simulink library "common_lib"  (R2021b)
settings: Solver=ode45  StartTime=0.0  StopTime=10.0  RelTol=1e-3
undefined symbols (not defined in the file or in its folder): ACCEL_PRE_MULT, C_C1GearNumbers, C_C1GearRatios, C_Calibration, C_DitherWaveform, C_GearOffset, C_GearRatioIn, C_GearRatioInverseOut, C_GearRatioOut, CLUTCH_INNER_LOOP_UPDATE_RATE, CONSTANT, DEGRADED_MODE_SIZE, Dem_EventStatusType, DiscIntNeverNeededParam, F_FAULT_ENUM, F_NOFAULT, F_OUTOFRANGE, F_RATELIMIT, FALSE, FMI14_SPECIAL_INSTRUCTIONS, FMI20_DATA_DRIFTED_HIGH, FMI21_DATA_DRIFTED_LOW, FMI29_RESERVED_FOR_SAE_ASSIGNMENT, FMI30_RESERVED_FOR_SAE_ASSIGNMENT, FMI31_CONDITION_EXISTS, FMI32_NO_FAULT, IC, k_accel, k_mean, LVDCU_OORH_FaultCntThd_C, MAX_UINT32, MEAN_PRE_MULT, NTriggers, QLTY_SIGNAL_FAILED, QLTY_SIGNAL_FULLY_FUNCTION, QLTY_SIGNAL_SUBSTITUTED_BY_1ST_CHOICE, QLTY_SIGNAL_SUBSTITUTED_BY_2ND_CHOICE, QLTY_SIGNAL_SUBSTITUTED_BY_3RD_CHOICE, QLTY_SIGNAL_SUBSTITUTED_BY_4TH_CHOICE, SAMPLE_TIME_100_mSec, SAMPLE_TIME_100_uSec, simin, T_TestPoint, TF_FALSE, TF_TRUE, TimeStep, TRUE, WORKSPACE_UPDATE_RATE, ZERO, Zero
libraries: $bdroot x120, simulink x27, simulink_extras x4, MBD_EPS_Local_Blockset x4
(part 8 of 10)

== system common_lib/Slink/Variable Rate Limiter ==
  note: Common Library::Simulink Enhancements::Rate Limiter
  input : Inport
  rise rate : Inport  Port=2
  fall rate : Inport  Port=3
  Data Type Conversion : DataTypeConversion  OutDataTypeStr=single
  Product : Product  InputSameDT=on  OutDataTypeStr=Inherit: Same as first input
  Product1 : Product  Inputs=/*  InputSameDT=on  OutDataTypeStr=Inherit: Same as first input
  Sat : $bdroot/Slink/Sat
  Sum2 : Sum  Inputs=|++  InputSameDT=on  OutDataTypeStr=Inherit: Same as first input
  Sum3 : Sum  Inputs=|+-  InputSameDT=on  OutDataTypeStr=Inherit: Same as first input
  T : Constant  Value=TimeStep
  Unit Delay : UnitDelay  InitialCondition=ic  SampleTime=-1  HasFrameUpgradeWarning=on
  output : Outport  VectorParamsAs1DForOutWhenUnconnected=off
  wires:
  Data Type Conversion/1 -> Product1/1, Product/1
  T/1 -> Data Type Conversion/1
  rise rate/1 -> Sat/2
  fall rate/1 -> Sat/3
  Sum3/1 -> Product1/2
  Product/1 -> Sum2/1
  Sum2/1 -> output/1, Unit Delay/1
  Unit Delay/1 -> Sum2/2, Sum3/2
  Product1/1 -> Sat/1  "Slope"
  input/1 -> Sum3/1
  Sat/1 -> Product/2

== system common_lib/Slink/Variable Rate Limiter w IC ==
  note: Common Library::Simulink Enhancements::Rate Limiter with Reset
  input : Inport
  rise rate : Inport  Port=2
  fall rate : Inport  Port=3
  ic : Inport  Port=4
  reset? : Inport  Port=5  OutDataTypeStr=boolean
  Data Type Conversion : DataTypeConversion  OutDataTypeStr=single
  Product : Product  InputSameDT=on  OutDataTypeStr=Inherit: Same as first input
  Product1 : Product  Inputs=/*  InputSameDT=on  OutDataTypeStr=Inherit: Same as first input
  Sat : $bdroot/Slink/Sat
  Sum2 : Sum  Inputs=|++  InputSameDT=on  OutDataTypeStr=Inherit: Same as first input
  Sum3 : Sum  Inputs=|+-  InputSameDT=on  OutDataTypeStr=Inherit: Same as first input
  Switch2 : Switch  Threshold=0.5  ZeroCross=off  InputSameDT=on
  T : Constant  Value=TimeStep
  Unit Delay1 : UnitDelay  InitialCondition=ic  SampleTime=-1  HasFrameUpgradeWarning=on
  output : Outport  VectorParamsAs1DForOutWhenUnconnected=off
  wires:
  Data Type Conversion/1 -> Product1/1, Product/1
  T/1 -> Data Type Conversion/1
  Switch2/1 -> Unit Delay1/1, output/1
  Sum2/1 -> Switch2/3
  Unit Delay1/1 -> Sum3/2, Sum2/2
  ic/1 -> Switch2/1
  reset?/1 -> Switch2/2
  Sat/1 -> Product/2
  input/1 -> Sum3/1
  Product1/1 -> Sat/1  "Slope"
  Product/1 -> Sum2/1
  Sum3/1 -> Product1/2
  fall rate/1 -> Sat/3
  rise rate/1 -> Sat/2

== system common_lib/Slink/Variable Rate Limiter w IC and Sat ==
  note: Common Library::Simulink Enhancements::Rate Limiter with Reset and Saturation
  input : Inport
  rise rate : Inport  Port=2
  fall rate : Inport  Port=3
  ulim : Inport  Port=4
  llim : Inport  Port=5
  ic : Inport  Port=6
  reset? : Inport  Port=7  OutDataTypeStr=boolean
  Data Type Conversion : DataTypeConversion  OutDataTypeStr=single
  Product : Product  InputSameDT=on  OutDataTypeStr=Inherit: Same as first input
  Product1 : Product  Inputs=/*  InputSameDT=on  OutDataTypeStr=Inherit: Same as first input
  Sat : $bdroot/Slink/Sat
  Sat1 : $bdroot/Slink/Sat
  Sum2 : Sum  Inputs=|++  InputSameDT=on  OutDataTypeStr=Inherit: Same as first input
  Sum3 : Sum  Inputs=|+-  InputSameDT=on  OutDataTypeStr=Inherit: Same as first input
  Switch2 : Switch  Threshold=0.5  ZeroCross=off  InputSameDT=on
  T : Constant  Value=TimeStep
  Unit Delay1 : UnitDelay  InitialCondition=ic  SampleTime=-1  HasFrameUpgradeWarning=on
  output : Outport  VectorParamsAs1DForOutWhenUnconnected=off
  wires:
  Data Type Conversion/1 -> Product1/1, Product/1
  T/1 -> Data Type Conversion/1
  llim/1 -> Sat1/3
  ulim/1 -> Sat1/2
  Switch2/1 -> Sat1/1
  Sat1/1 -> Unit Delay1/1, output/1
  Sum2/1 -> Switch2/3
  Unit Delay1/1 -> Sum3/2, Sum2/2
  ic/1 -> Switch2/1
  reset?/1 -> Switch2/2
  Sat/1 -> Product/2
  input/1 -> Sum3/1
  Product1/1 -> Sat/1  "Slope"
  Product/1 -> Sum2/1
  Sum3/1 -> Product1/2
  fall rate/1 -> Sat/3
  rise rate/1 -> Sat/2

== system common_lib/Tbl/2D Lookup ==
  Input : Inport
  X Axis : Inport  Port=2
  Y Axis : Inport  Port=3
  Mux : Mux  Inputs=3
  S-Function : S-Function  FunctionName=vartable  Parameters=Mode  SFunctionDeploymentMode=off  EnableBusSupport=off
  Output : Outport  VectorParamsAs1DForOutWhenUnconnected=off
  wires:
  Mux/1 -> S-Function/1
  Input/1 -> Mux/1
  X Axis/1 -> Mux/2
  S-Function/1 -> Output/1
  Y Axis/1 -> Mux/3

== system common_lib/Tbl/Interpolator ==
  note: Common Library::Tables::Interpolator
  value_1 : Inport
  value_0 : Inport  Port=2
  interp_factor : Inport  Port=3
  Constant1 : Constant  Value=Zero
  Constant2 : Constant  Value=One
  XY Interpolator : $bdroot/Tbl/XY Interpolator  DType=double
  output : Outport  VectorParamsAs1DForOutWhenUnconnected=off
  wires:
  value_0/1 -> XY Interpolator/2
  value_1/1 -> XY Interpolator/1
  Constant2/1 -> XY Interpolator/3
  Constant1/1 -> XY Interpolator/4
  interp_factor/1 -> XY Interpolator/5
  XY Interpolator/1 -> output/1

== system common_lib/Tbl/XY Interpolator ==
  note: Common Library::Tables::XY Interpolator
  y_value_1 : Inport
  y_value_0 : Inport  Port=2
  x_value_1 : Inport  Port=3
  x_value_0 : Inport  Port=4
  x_value : Inport  Port=5
  Interp : S-Function  FunctionName=xyinterp_f32_wrap  SFunctionModules=xyinterp_f32  SFunctionDeploymentMode=off  EnableBusSupport=off
  output : Outport  VectorParamsAs1DForOutWhenUnconnected=off
  wires:
  y_value_1/1 -> Interp/1
  y_value_0/1 -> Interp/2
  x_value_1/1 -> Interp/3
  x_value_0/1 -> Interp/4
  x_value/1 -> Interp/5
  Interp/1 -> output/1

== system common_lib/Tbl/XY Interpolator1 ==
  note: Common Library::Tables::XY Interpolator
  y_value_1 : Inport
  y_value_0 : Inport  Port=2
  x_value_1 : Inport  Port=3
  x_value_0 : Inport  Port=4
  x_value : Inport  Port=5
  DTC{,1..4} (5 alike) : DataTypeConversion  OutDataTypeStr=single
  Signal Conversion : SignalConversion  ConversionOutput=Contiguous copy  OverrideOpt=on
  XYInterp : Subsystem  TreatAsAtomicUnit=on  RTWFcnName=XYINT
      settings: RTWFcnNameOpts=User specified  RTWFileNameOpts=Use function name
  output : Outport  VectorParamsAs1DForOutWhenUnconnected=off
  wires:
  Signal Conversion/1 -> output/1
  DTC4/1 -> XYInterp/5(x_value)
  DTC3/1 -> XYInterp/4(x_value_0)
  DTC2/1 -> XYInterp/3(x_value_1)
  DTC1/1 -> XYInterp/2(y_value_0)
  DTC/1 -> XYInterp/1(y_value_1)
  x_value/1 -> DTC4/1
  x_value_0/1 -> DTC3/1
  x_value_1/1 -> DTC2/1
  XYInterp/1(output) -> Signal Conversion/1
  y_value_0/1 -> DTC1/1
  y_value_1/1 -> DTC/1

== system common_lib/Timers/Timer ==
  In : Inport
  TriggerTime : Inport  Port=2
  Data Type Conversion : DataTypeConversion  OutDataTypeStr=single
  Discrete-Time Integrator : DiscreteIntegrator  gainval=single(1.0)  ExternalReset=falling  InitialCondition=single(0)  SampleTime=TimeStep  LimitOutput=on  ICPrevOutput=DiscIntNeverNeededParam  ICPrevScaledInput=DiscIntNeverNeededParam
  Relational Operator : RelationalOperator  Operator=>  OutDataTypeStr=boolean  RndMeth=Nearest
  Signal Specification : SignalSpecification  OutDataTypeStr=boolean
  Out : Outport  VectorParamsAs1DForOutWhenUnconnected=off
  wires:
  Signal Specification/1 -> Discrete-Time Integrator/2, Data Type Conversion/1
  In/1 -> Signal Specification/1
  Data Type Conversion/1 -> Discrete-Time Integrator/1
  Discrete-Time Integrator/1 -> Relational Operator/1
  TriggerTime/1 -> Relational Operator/2
  Relational Operator/1 -> Out/1

== system common_lib/Approved Simulink/Basic IO/M_MonitorParameter1 ==
  Input : Inport
  towork : ToWorkspace  VariableName=ToWorkspace  SampleTime=-1
      settings: Description=Monitor  Decimation=WORKSPACE_DECIMATION
  wires:
  Input/1 -> towork/1  "ToWorkspace"

== system common_lib/Approved Simulink/Basic IO/To xPC Scope1 ==
  Inport : Inport
  Terminate : Terminator
  wires:
  Inport/1 -> Terminate/1

== system common_lib/Approved Simulink/SubSys Triggers/Configurable Subsystem ==

== system common_lib/Approved Simulink/SubSys Triggers/For Iterator Subsystem ==
  In1 : Inport
  For Iterator : ForIterator
  Out1 : Outport  VectorParamsAs1DForOutWhenUnconnected=off
  wires:
  In1/1 -> Out1/1

== system common_lib/Approved Simulink/SubSys Triggers/If Action Subsystem ==
  In1 : Inport
  Action Port : ActionPort
  Out1 : Outport  VectorParamsAs1DForOutWhenUnconnected=off
  wires:
  In1/1 -> Out1/1

== system common_lib/Approved Simulink/SubSys Triggers/Subsystem ==
  In1 : Inport
  Out1 : Outport  VectorParamsAs1DForOutWhenUnconnected=off
  wires:
  In1/1 -> Out1/1

== system common_lib/Approved Simulink/SubSys Triggers/While Iterator Subsystem ==
  In1 : Inport
  IC : Inport  Port=2
  While Iterator : WhileIterator
  Out1 : Outport  VectorParamsAs1DForOutWhenUnconnected=off
  wires:
  IC/1 -> While Iterator/2
  In1/1 -> Out1/1

== system common_lib/Ctrl/DTNA_PIgov/Integrator ==
  note: Common Library::Integral
  input : Inport
  ulim : Inport  Port=2
  llim : Inport  Port=3
  ic : Inport  Port=4
  reset? : Inport  Port=5  OutDataTypeStr=boolean
  Constant1 : Constant  Value=TimeStep  OutDataTypeStr=Inherit: Inherit via back propagation
  Product1 : Product  Inputs=**  InputSameDT=on  OutDataTypeStr=Inherit: Same as first input
  Sat : Subsystem  AncestorBlock=common_lib/Slink/Sat  mask(CL Variable Saturation){}
      mask help:
      | Variable saturation block
      |
      | X(1) = input
      | X(2) = upper limit
      | X(3) = lower limit
      |
      | Y(1) = output
      | NgEK, Inc.
      mask Help: web(which(['common_lib37.html']))
      mask Display:
      | patch([0.3 0.3 0.7 0.7], [0.35 0.65 0.65 0.35], [255/255 127/255 255/255])
      | 
      | plot([0 1],[0.5 0.5],[0.5 0.5],[0 1],[0 0.25 0.75 1],[0 0 1 1])
  Sum : Sum  Inputs=++|  InputSameDT=on  OutDataTypeStr=Inherit: Same as first input
  Switch : Switch  Threshold=0.5  ZeroCross=off  InputSameDT=on
  Unit Delay : UnitDelay  InitialCondition=IC  SampleTime=-1  HasFrameUpgradeWarning=on
  Output : Outport  VectorParamsAs1DForOutWhenUnconnected=off
  wires:
  Constant1/1 -> Product1/1
  Sat/1(output) -> Unit Delay/1, Output/1
  Unit Delay/1 -> Sum/1
  Switch/1 -> Sat/1(input)
  Sum/1 -> Switch/3
  llim/1 -> Sat/3(llim)
  ulim/1 -> Sat/2(ulim)
  reset?/1 -> Switch/2
  Product1/1 -> Sum/2
  ic/1 -> Switch/1
  input/1 -> Product1/2

== system common_lib/Ctrl/Derivative/DerivativeCoreLogic ==
  note: s
      | H(s) = ----------------
      |              1+s/Klo
  note: Derivative Filter Obtained By Backward Differencing Of
  input : Inport  OutDataTypeStr=single
  cutoff : Inport  Port=2  OutDataTypeStr=single
  reset? : Inport  Port=3  OutDataTypeStr=boolean
  ulim : Inport  Port=4
  llim : Inport  Port=5
  Constant1 : Constant  Value=One
  Constant6 : Constant  Value=Zero
  IC:  0 : UnitDelay  InitialCondition=Zero  SampleTime=-1  HasFrameUpgradeWarning=on
  IC: 0 : UnitDelay  InitialCondition=Zero  SampleTime=-1  HasFrameUpgradeWarning=on
  Product2 : Product  Inputs=*/  InputSameDT=on  OutDataTypeStr=Inherit: Same as first input
  Sat : $bdroot/Slink/Sat
  Sum : Sum  Inputs=++-  InputSameDT=on  OutDataTypeStr=Inherit: Same as first input
  Sum3 : Sum  Inputs=|++  InputSameDT=on  OutDataTypeStr=Inherit: Same as first input
  Switch : Switch  Criteria=u2 ~= 0  Threshold=0.5  ZeroCross=off  InputSameDT=on
  output : Outport  OutDataTypeStr=single  VectorParamsAs1DForOutWhenUnconnected=off
  wires:
  reset?/1 -> Switch/2
  Switch/1 -> IC: 0/1, Sat/1
  Constant6/1 -> Switch/1
  Product2/1 -> Switch/3
  IC: 0/1 -> Sum/1
  Sum3/1 -> Product2/2
  Constant1/1 -> Sum3/2
  IC:  0/1 -> Sum/3
  input/1 -> IC:  0/1, Sum/2
  cutoff/1 -> Sum3/1
  Sum/1 -> Product2/1
  ulim/1 -> Sat/2
  llim/1 -> Sat/3
  Sat/1 -> output/1

== system common_lib/Ctrl/PIgov/Integrator01 ==
  note: Common Library::Integral
  input : Inport
  ulim : Inport  Port=2
  llim : Inport  Port=3
  ic : Inport  Port=4
  reset? : Inport  Port=5  OutDataTypeStr=boolean
  Constant1 : Constant  Value=TimeStep
  Product1 : Product  Inputs=**  InputSameDT=on  OutDataTypeStr=Inherit: Same as first input
  Sat : $bdroot/Slink/Sat
  Sum : Sum  Inputs=++|  InputSameDT=on  OutDataTypeStr=Inherit: Same as first input
  Switch : Switch  Threshold=0.5  ZeroCross=off  InputSameDT=on
  Unit Delay : UnitDelay  InitialCondition=IC  SampleTime=-1  HasFrameUpgradeWarning=on
  Output : Outport  VectorParamsAs1DForOutWhenUnconnected=off
  wires:
  Constant1/1 -> Product1/1
  Sat/1 -> Unit Delay/1, Output/1
  Unit Delay/1 -> Sum/1
  Switch/1 -> Sat/1
  Sum/1 -> Switch/3
  llim/1 -> Sat/3
  ulim/1 -> Sat/2
  reset?/1 -> Switch/2
  Product1/1 -> Sum/2
  ic/1 -> Switch/1
  input/1 -> Product1/2

== system common_lib/Ctrl/Trajectory/CurrentStart ==
  in : Inport
  Enable : EnablePort  ZeroCross=off
  out : Outport  VectorParamsAs1DForOutWhenUnconnected=off
  wires:
  in/1 -> out/1

== system common_lib/Ctrl/Trajectory/Start ==
  in : Inport
  Enable : EnablePort  ZeroCross=off
  out : Outport  VectorParamsAs1DForOutWhenUnconnected=off
  wires:
  in/1 -> out/1

== system common_lib/Ctrl/Trajectory/Variable Rate Limiter w IC in feedback loop ==
  note: Common Library::Simulink Enhancements::Rate Limiter with IC in feedback loop
  input : Inport
  rise rate : Inport  Port=2
  fall rate : Inport  Port=3
  ic : Inport  Port=4
  reset? : Inport  Port=5  OutDataTypeStr=boolean
  Product : Product  InputSameDT=on  OutDataTypeStr=Inherit: Same as first input
  Product1 : Product  Inputs=/*  InputSameDT=on  OutDataTypeStr=Inherit: Same as first input
  Sat : $bdroot/Slink/Sat
  Sum2 : Sum  Inputs=|++  InputSameDT=on  OutDataTypeStr=Inherit: Same as first input
  Sum3 : Sum  Inputs=|+-  InputSameDT=on  OutDataTypeStr=Inherit: Same as first input
  Switch2 : Switch  Threshold=0.5  ZeroCross=off  InputSameDT=on
  T : Constant  Value=TimeStep
  Unit Delay1 : UnitDelay  InitialCondition=ic  SampleTime=-1  HasFrameUpgradeWarning=on
  output : Outport  VectorParamsAs1DForOutWhenUnconnected=off
  wires:
  Switch2/1 -> Sum2/2, Sum3/2
  input/1 -> Sum3/1
  Sum2/1 -> Unit Delay1/1, output/1
  Unit Delay1/1 -> Switch2/3
  ic/1 -> Switch2/1
  reset?/1 -> Switch2/2
  Sat/1 -> Product/2
  Product1/1 -> Sat/1  "Slope"
  Product/1 -> Sum2/1
  Sum3/1 -> Product1/2
  T/1 -> Product1/1, Product/1
  fall rate/1 -> Sat/3
  rise rate/1 -> Sat/2

== system common_lib/Diag/Command Feedback Test/CommandFeedbackFaultLogicCore ==
  note: Check for command-feedback error exceeding threshold.
  note: Check for "steady state"
  cmd : Inport  OutDataTypeStr=single
  fbk : Inport  Port=2  OutDataTypeStr=single
  tau : Inport  Port=3  OutDataTypeStr=single
  tau_lim : Inport  Port=4  OutDataTypeStr=single
  tau_time : Inport  Port=5  OutDataTypeStr=single
  error_lim : Inport  Port=6  OutDataTypeStr=single
  error_time : Inport  Port=7  OutDataTypeStr=single
  Abs : Abs  ZeroCross=off
  Abs2 : Abs  ZeroCross=off
  Constant1 : Constant  Value=Zero
  Constant3 : Constant  Value=Zero
  Constant5 : Constant  Value=MinusOne
  EdgeTriggered Pulse w/time1 : $bdroot/Misc/EdgeTriggered Pulse w time  Edge=TRUE to FALSE  Pulse=TRUE  TimeStep=TimeStep  Init=0
  Fltr : $bdroot/Fltrs/Fltr  TimeStep=TimeStep
  Latch : $bdroot/Misc/Latch  IC=false
  Logical Operator1 : Logic  Operator=OR
  Product2 : Product  InputSameDT=on  OutDataTypeStr=Inherit: Same as first input
  Relational Operator1 : RelationalOperator  ZeroCross=off  RndMeth=Nearest  InputSameDT=on
  Relational Operator2 : RelationalOperator  ZeroCross=off  RndMeth=Nearest  InputSameDT=on
  Relational Operator3 : RelationalOperator  ZeroCross=off  RndMeth=Nearest  InputSameDT=on
  Relational Operator4 : RelationalOperator  Operator=<=  ZeroCross=off  RndMeth=Nearest  InputSameDT=on
  Sat : $bdroot/Slink/Sat
  Sum : Sum  Inputs=|+-  InputSameDT=on  OutDataTypeStr=Inherit: Same as first input
  Sum2 : Sum  Inputs=|+-  InputSameDT=on  OutDataTypeStr=Inherit: Same as first input
  Sum3 : Sum  Inputs=++|  InputSameDT=on  OutDataTypeStr=Inherit: Same as first input
  T1 : Constant  Value=Ts
  Unit Delay1 : UnitDelay  InitialCondition=Zero  SampleTime=-1  HasFrameUpgradeWarning=on
  dec switch : Switch  Threshold=0.5  ZeroCross=off  InputSameDT=on
  dec switch1 : Switch  Threshold=0.5  ZeroCross=off  InputSameDT=on
  Min Value : Outport  OutDataTypeStr=boolean  VectorParamsAs1DForOutWhenUnconnected=off
  wires:
  T1/1 -> Product2/1, dec switch1/1
  Product2/1 -> dec switch1/3
  Constant5/1 -> Product2/2
  Relational Operator4/1 -> Latch/2
  Relational Operator3/1 -> Latch/1
  Latch/1 -> Min Value/1
  Logical Operator1/1 -> dec switch/2
  Relational Operator2/1 -> dec switch1/2
  Constant1/1 -> dec switch/1
  dec switch1/1 -> dec switch/3
  Unit Delay1/1 -> Sum3/1
  Sat/1 -> Unit Delay1/1
  dec switch/1 -> Sum3/2
  Constant3/1 -> Relational Operator4/2, Sat/3
  error_time/1 -> Relational Operator3/2, Sat/2
  Sum3/1 -> Relational Operator4/1, Relational Operator3/1, Sat/1
  error_lim/1 -> Relational Operator2/2
  Abs/1 -> Relational Operator2/1
  EdgeTriggered Pulse w/time1/1 -> Logical Operator1/2
  tau_time/1 -> EdgeTriggered Pulse w/time1/2
  Relational Operator1/1 -> Logical Operator1/1, EdgeTriggered Pulse w/time1/1
  tau_lim/1 -> Relational Operator1/2
  Abs2/1 -> Relational Operator1/1
  Sum2/1 -> Abs2/1
  tau/1 -> Fltr/2
  Fltr/1 -> Sum2/2
  Sum/1 -> Abs/1
  fbk/1 -> Sum/2
  cmd/1 -> Sum2/1, Fltr/1, Sum/1

== system common_lib/Diag/Fault Counter/FaultCounter ==
  fl : Inport
  count_prev : Inport  Port=2
  fc_level : Inport  Port=3
  reset : Inport  Port=4  OutDataTypeStr=boolean
  Enable : EnablePort  ZeroCross=off
  Constant1 : Constant  Value=ZERO
  Constant2 : Constant  Value=false
  Constant3 : Constant  Value=true
  Constant6 : Constant  Value=ZERO
  Relay : $bdroot/Slink/Relay  init=false
      settings: AttributesFormatString=ic=%<init>
  Sat : $bdroot/Slink/Sat
  Sum : Sum  Inputs=++|  InputSameDT=on  OutDataTypeStr=Inherit: Same as first input
  reset switch1 : Switch  Criteria=u2 ~= 0  Threshold=0.5  ZeroCross=off  InputSameDT=on
  count : Outport  OutputWhenDisabled=reset  InitialOutput=ZERO  VectorParamsAs1DForOutWhenUnconnected=off
  fc : Outport  Port=2  OutputWhenDisabled=reset  InitialOutput=false  VectorParamsAs1DForOutWhenUnconnected=off
  wires:
  Sum/1 -> reset switch1/3
  Constant6/1 -> reset switch1/1
  Relay/1 -> fc/1
  Constant3/1 -> Relay/4
  Constant2/1 -> Relay/5
  Constant1/1 -> Relay/3, Sat/3
  fc_level/1 -> Relay/2, Sat/2
  fl/1 -> Sum/2
  reset/1 -> reset switch1/2
  reset switch1/1 -> Relay/1, Sat/1
  count_prev/1 -> Sum/1
  Sat/1 -> count/1

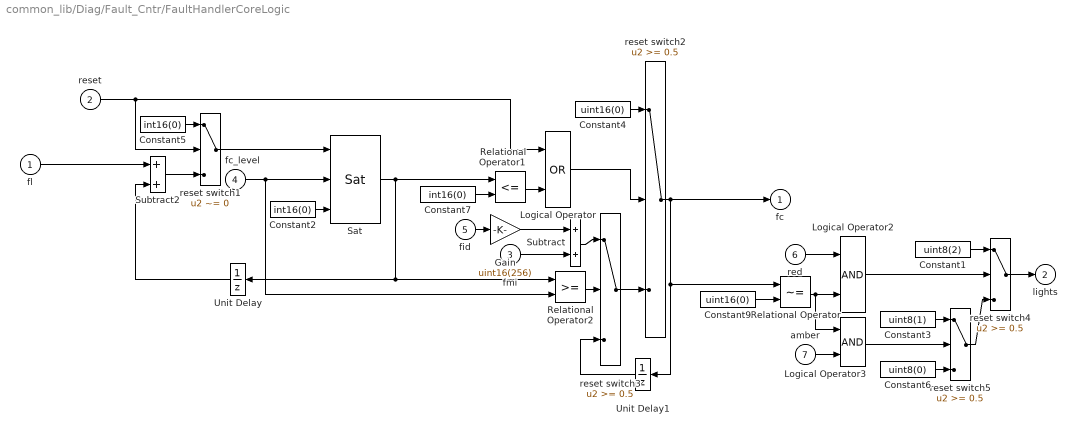
== system common_lib/Diag/Fault_Cntr/FaultHandlerCoreLogic ==
  fl : Inport  OutDataTypeStr=int16
  reset : Inport  Port=2  OutDataTypeStr=boolean
  fmi : Inport  Port=3  OutDataTypeStr=uint16
  fc_level : Inport  Port=4  OutDataTypeStr=int16
  fid : Inport  Port=5  OutDataTypeStr=uint16
  red : Inport  Port=6  OutDataTypeStr=boolean
  amber : Inport  Port=7  OutDataTypeStr=boolean
  Constant1 : Constant  Value=uint8(2)
  Constant2 : Constant  Value=int16(0)
  Constant3 : Constant  Value=uint8(1)
  Constant4 : Constant  Value=uint16(0)
  Constant5 : Constant  Value=int16(0)
  Constant6 : Constant  Value=uint8(0)
  Constant7 : Constant  Value=int16(0)
  Constant9 : Constant  Value=uint16(0)
  Gain : Gain  Gain=uint16(256)
  Logical Operator : Logic  Operator=OR  AllPortsSameDT=off  OutDataTypeStr=boolean
  Logical Operator2 : Logic  AllPortsSameDT=off  OutDataTypeStr=boolean
  Logical Operator3 : Logic  AllPortsSameDT=off  OutDataTypeStr=boolean
  Relational Operator : RelationalOperator  Operator=~=  OutDataTypeStr=boolean  RndMeth=Nearest
  Relational Operator1 : RelationalOperator  Operator=<=  OutDataTypeStr=boolean  RndMeth=Nearest
  Relational Operator2 : RelationalOperator  OutDataTypeStr=boolean  RndMeth=Nearest
  Sat : $bdroot/Slink/Sat
  Subtract : Sum  OutDataTypeStr=uint16
  Subtract2 : Sum  OutDataTypeStr=int16  SaturateOnIntegerOverflow=on
  Unit Delay : UnitDelay  InitialCondition=int16(0)  SampleTime=-1  HasFrameUpgradeWarning=on
      settings: AttributesFormatString=ic=%<X0>
  Unit Delay1 : UnitDelay  InitialCondition=uint16(0)  SampleTime=-1  HasFrameUpgradeWarning=on
      settings: AttributesFormatString=ic=%<X0>
  reset switch1 : Switch  Criteria=u2 ~= 0  Threshold=0.5  ZeroCross=off  InputSameDT=on
  reset switch{2..5} (4 alike) : Switch  Threshold=0.5  ZeroCross=off  InputSameDT=on
  fc : Outport  VectorParamsAs1DForOutWhenUnconnected=off
  lights : Outport  Port=2  VectorParamsAs1DForOutWhenUnconnected=off
  wires:
  Gain/1 -> Subtract/1
  reset switch3/1 -> reset switch2/3
  Unit Delay1/1 -> reset switch3/3
  Relational Operator2/1 -> reset switch3/2
  Relational Operator1/1 -> Logical Operator/2
  Constant7/1 -> Relational Operator1/2
  Unit Delay/1 -> Subtract2/2
  Subtract2/1 -> reset switch1/3
  reset switch1/1 -> Sat/1
  Constant5/1 -> reset switch1/1
  reset switch2/1 -> Unit Delay1/1, Relational Operator/1, fc/1
  Logical Operator/1 -> reset switch2/2
  Subtract/1 -> reset switch3/1
  Constant4/1 -> reset switch2/1
  fmi/1 -> Subtract/2
  fid/1 -> Gain/1
  reset/1 -> Logical Operator/1, reset switch1/2
  fl/1 -> Subtract2/1
  Sat/1 -> Relational Operator2/1, Unit Delay/1, Relational Operator1/1
  Constant9/1 -> Relational Operator/2
  Logical Operator2/1 -> reset switch4/2
  Relational Operator/1 -> Logical Operator2/2, Logical Operator3/1
  red/1 -> Logical Operator2/1
  amber/1 -> Logical Operator3/2
  fc_level/1 -> Sat/2, Relational Operator2/2
  Constant2/1 -> Sat/3
  Constant1/1 -> reset switch4/1
  Logical Operator3/1 -> reset switch5/2
  reset switch5/1 -> reset switch4/3
  Constant3/1 -> reset switch5/1
  Constant6/1 -> reset switch5/3
  reset switch4/1 -> lights/1

== system common_lib/Diag/Filter w Fault Handler/FilterWithFaultHandlerCoreLogic ==
  note: Common Library::Diagnostics::Filter With Fault Handler
  input : Inport
  tau : Inport  Port=2
  override_value : Inport  Port=3
  override? : Inport  Port=4
  reset? : Inport  Port=5
  default : Inport  Port=6
  ramp_time : Inport  Port=7
  fault? : Inport  Port=8
  Abs1 : Abs  ZeroCross=off
  Abs2 : Abs  ZeroCross=off
  Constant5 : Constant  Value=TimeStep
  Data Type Conversion : DataTypeConversion  OutDataTypeStr=single
  Fltr_wRO : $bdroot/Fltrs/Fltr_wRO  TimeStep=TimeStep
  Product1 : Product  Inputs=**/  InputSameDT=on  OutDataTypeStr=Inherit: Same as first input
  Sum1 : Sum  Inputs=+-|  InputSameDT=on  OutDataTypeStr=Inherit: Same as first input
  Sum2 : Sum  Inputs=+-|  InputSameDT=on  OutDataTypeStr=Inherit: Same as first input
  Sum3 : Sum  Inputs=+-|  InputSameDT=on  OutDataTypeStr=Inherit: Same as first input
  Switch{1..4} (4 alike) : Switch  Threshold=0.5  ZeroCross=off  InputSameDT=on
  delay : UnitDelay  InitialCondition=Zero  SampleTime=-1  HasFrameUpgradeWarning=on
  ic: signal at fault : UnitDelay  InitialCondition=Zero  SampleTime=-1  HasFrameUpgradeWarning=on
  within zero tol of corrections : RelationalOperator  Operator=<  ZeroCross=off  RndMeth=Nearest
  output : Outport  VectorParamsAs1DForOutWhenUnconnected=off
  wires:
  Data Type Conversion/1 -> Product1/2
  Constant5/1 -> Data Type Conversion/1
  Sum3/1 -> Abs1/1
  delay/1 -> Switch2/1
  Switch3/1 -> delay/1
  within zero tol of corrections/1 -> Switch3/2
  Abs2/1 -> within zero tol of corrections/1
  Abs1/1 -> within zero tol of corrections/2
  Sum2/1 -> Switch3/1
  Switch1/1 -> Sum3/1, Sum2/1
  Switch4/1 -> Switch1/3, Sum1/1, ic: signal at fault/1
  ic: signal at fault/1 -> Switch4/1
  Product1/1 -> Abs2/1, Sum2/2
  Sum1/1 -> Product1/1
  default/1 -> Sum3/2, Switch3/3, Sum1/2
  Fltr_wRO/1 -> Switch4/3, output/1
  input/1 -> Switch2/3
  Switch2/1 -> Switch1/1, Fltr_wRO/1
  reset?/1 -> Fltr_wRO/5
  override?/1 -> Fltr_wRO/4
  override_value/1 -> Fltr_wRO/3
  tau/1 -> Fltr_wRO/2
  fault?/1 -> Switch1/2, Switch4/2, Switch2/2
  ramp_time/1 -> Product1/3

== system common_lib/Diag/Filter w Fault Handler1/Fltr_wRO ==
  note: This is a simple 1st order filter block with reset and override.
      |
      |      If override is true (1) then output=override_value
      |      If       reset is true (1) then output=input
      |    otherwise output = previous output + (input - previous output) * T/tau
  note: Common Library::Filters::Filter with Reset and Override
  input : Inport
  tau : Inport  Port=2
  reset? : Inport  Port=3  OutDataTypeStr=boolean
  Constant1 : Constant  Value=TimeStep
  Constant3 : Constant  Value=TimeStep
  MinMax : MinMax  Function=max  Inputs=2  InputSameDT=on  SaturateOnIntegerOverflow=on  ZeroCross=off
  Product : Product  Inputs=**/  InputSameDT=on  OutDataTypeStr=Inherit: Same as first input
  Sum : Sum  Inputs=|+-  InputSameDT=on  OutDataTypeStr=Inherit: Same as first input
  Sum1 : Sum  Inputs=|++  InputSameDT=on  OutDataTypeStr=Inherit: Same as first input
  Switch2 : Switch  Threshold=0.5  ZeroCross=off  InputSameDT=on
  Unit Delay : UnitDelay  InitialCondition=IC  SampleTime=-1  HasFrameUpgradeWarning=on
  output : Outport  VectorParamsAs1DForOutWhenUnconnected=off
  wires:
  Sum1/1 -> Switch2/3
  Product/1 -> Sum1/1
  tau/1 -> MinMax/2
  Constant1/1 -> MinMax/1
  Unit Delay/1 -> Sum1/2, Sum/2
  input/1 -> Switch2/1, Sum/1
  Constant3/1 -> Product/2
  MinMax/1 -> Product/3
  reset?/1 -> Switch2/2
  Sum/1 -> Product/1
  Switch2/1 -> Unit Delay/1, output/1

== system common_lib/Diagnostics/Calibration Enabled Debounce Boolean Input/DiagFaultCounter ==
  diagFaultActive : Inport
  diagStartUpComp : Inport  Port=2
  diagReset : Inport  Port=3
  diagEnable : Inport  Port=4
  diagDbncEnab : Inport  Port=5
  diagFaultCntThresh : Inport  Port=6
  diagPassCntThresh : Inport  Port=7
  diagUpCnt : Inport  Port=8
  diagDnCnt : Inport  Port=9
  diagHealEn : Inport  Port=10
  DiagFaulCounter : Stateflow chart  TreatAsAtomicUnit=on
  diagFaultStatus : Outport  OutputWhenDisabled=reset  InitialOutput=Dem_EventStatusType.DEM_EVENT_STATUS_INIT  VectorParamsAs1DForOutWhenUnconnected=off
  diagFaultCnt : Outport  Port=2  OutputWhenDisabled=reset  InitialOutput=Dem_EventStatusType.DEM_EVENT_STATUS_INIT  VectorParamsAs1DForOutWhenUnconnected=off
  wires:
  diagFaultActive/1 -> DiagFaulCounter/1(diagFaultActive)
  diagFaultCntThresh/1 -> DiagFaulCounter/6(diagFaultCntThresh)
  diagReset/1 -> DiagFaulCounter/3(diagReset)
  diagUpCnt/1 -> DiagFaulCounter/8(diagUpCnt)
  diagDnCnt/1 -> DiagFaulCounter/9(diagDnCnt)
  diagEnable/1 -> DiagFaulCounter/4(diagEnable)
  DiagFaulCounter/1(diagFaultStatus) -> diagFaultStatus/1
  diagDbncEnab/1 -> DiagFaulCounter/5(diagDbncEnab)
  diagStartUpComp/1 -> DiagFaulCounter/2(diagStartUpComp)
  diagPassCntThresh/1 -> DiagFaulCounter/7(diagPassCntThresh)
  diagHealEn/1 -> DiagFaulCounter/10(diagHealEn)
  DiagFaulCounter/2(diagFaultCnt) -> diagFaultCnt/1

== system common_lib/Diagnostics/Calibration Enabled MinMax OOR/Enabled OOR ==
  In : Inport
  ULim : Inport  Port=2
  LLim : Inport  Port=3
  Ext_Fault : Inport  Port=4
  Enable : EnablePort  ZeroCross=off
      settings: AttributesFormatString=%<StatesWhenEnabling>
  Calibration with Pretty Print Value : $bdroot/IO/Calibration with Pretty Print Value  CalValue=C_IMgmt_OOR_MinMaxCapture_Enable  scaling=None
  OOR Fault Detection : $bdroot/Diag/OOR Fault Detection  InitialValue=InitialValue
  OOR MinMax Capture : Subsystem
  Out : Outport  InitialOutput=0  VectorParamsAs1DForOutWhenUnconnected=off
      settings: AttributesFormatString=|
      | OutputWhenDisabled=%<OutputWhenDisabled>
      | InitialOutput=%<InitialOutput>
  Fault : Outport  Port=2  InitialOutput=0  VectorParamsAs1DForOutWhenUnconnected=off
      settings: AttributesFormatString=|
      | OutputWhenDisabled=%<OutputWhenDisabled>
      | InitialOutput=%<InitialOutput>
  Max : Outport  Port=3  VectorParamsAs1DForOutWhenUnconnected=off
      settings: AttributesFormatString=|
      | OutputWhenDisabled=%<OutputWhenDisabled>
      | InitialOutput=%<InitialOutput>
  Min : Outport  Port=4  VectorParamsAs1DForOutWhenUnconnected=off
      settings: AttributesFormatString=|
      | OutputWhenDisabled=%<OutputWhenDisabled>
      | InitialOutput=%<InitialOutput>
  wires:
  LLim/1 -> OOR Fault Detection/3
  ULim/1 -> OOR Fault Detection/2
  In/1 -> OOR Fault Detection/1, OOR MinMax Capture/1(Input)
  Ext_Fault/1 -> OOR Fault Detection/4, OOR MinMax Capture/2(Hold)
  OOR Fault Detection/1 -> Out/1
  OOR Fault Detection/2 -> Fault/1
  OOR MinMax Capture/1(Max) -> Max/1
  OOR MinMax Capture/2(Min) -> Min/1
  Calibration with Pretty Print Value/1 -> OOR MinMax Capture/Enable

== system common_lib/Diagnostics/Calibration Enabled MinMax RLim/Enabled RLim ==
  In : Inport
  RLim : Inport  Port=2
  Ext_Fault : Inport  Port=3
  Enable : EnablePort  ZeroCross=off
      settings: AttributesFormatString=%<StatesWhenEnabling>
  Calibration with Pretty Print Value : $bdroot/IO/Calibration with Pretty Print Value  CalValue=C_IMgmt_RLim_MinMaxCapture_Enable  scaling=None
  Data Type Conversion : DataTypeConversion  OutDataTypeStr=single
  Data Type Conversion1 : DataTypeConversion  OutDataTypeStr=single
  RLim MinMax Capture : Subsystem
  RateLimit : Subsystem  mask{IC=IC, TimeStep=TimeStep}
      mask prompts: IC "Initial Condition"; TimeStep "Update Time"
  out : Outport  VectorParamsAs1DForOutWhenUnconnected=off
      settings: AttributesFormatString=|
      | OutputWhenDisabled=%<OutputWhenDisabled>
      | InitialOutput=%<InitialOutput>
  fault? : Outport  Port=2  VectorParamsAs1DForOutWhenUnconnected=off
      settings: AttributesFormatString=|
      | OutputWhenDisabled=%<OutputWhenDisabled>
      | InitialOutput=%<InitialOutput>
  Max Pos Rate : Outport  Port=3  VectorParamsAs1DForOutWhenUnconnected=off
      settings: AttributesFormatString=|
      | OutputWhenDisabled=%<OutputWhenDisabled>
      | InitialOutput=%<InitialOutput>
  Max Neg Rate : Outport  Port=4  VectorParamsAs1DForOutWhenUnconnected=off
      settings: AttributesFormatString=|
      | OutputWhenDisabled=%<OutputWhenDisabled>
      | InitialOutput=%<InitialOutput>
  wires:
  In/1 -> Data Type Conversion/1, RLim MinMax Capture/1(Input)
  Ext_Fault/1 -> RLim MinMax Capture/2(Hold), RateLimit/3(ext_fault?)
  RateLimit/1(out) -> out/1
  RLim/1 -> Data Type Conversion1/1
  RateLimit/2(fault?) -> fault?/1
  RLim MinMax Capture/2(Min) -> Max Neg Rate/1
  RLim MinMax Capture/1(Max) -> Max Pos Rate/1
  Data Type Conversion/1 -> RateLimit/1(in)
  Data Type Conversion1/1 -> RateLimit/2(rlim)
  Calibration with Pretty Print Value/1 -> RLim MinMax Capture/Enable

== system common_lib/Diagnostics/DTNA_Diag/CC_Diag ==
  diagInput : Inport
  diagStartUpComp : Inport  Port=2
  diagUpCnt : Inport  Port=3
  diagDnCnt : Inport  Port=4
  diagFaultCntThresh : Inport  Port=5
  diagPassCntThresh : Inport  Port=6
  diagDbncEnab : Inport  Port=7
  diagReset : Inport  Port=8
  diagEnable : Inport  Port=9
  diagHealEn : Inport  Port=10
  Ccaller_DiagLv1 : Subsystem  AncestorBlock=common_lib/Diagnostics/Ccaller_DiagLv1  TreatAsAtomicUnit=on
      settings: RTWSystemCode=Nonreusable function
  diagFaultStatus : Outport
  diagFaultCnt : Outport  Port=2
  wires:
  diagInput/1 -> Ccaller_DiagLv1/1(diagFaultActive)
  diagStartUpComp/1 -> Ccaller_DiagLv1/2(diagStartUpComp)
  diagUpCnt/1 -> Ccaller_DiagLv1/8(diagUpCnt)
  diagDnCnt/1 -> Ccaller_DiagLv1/9(diagDnCnt)
  diagFaultCntThresh/1 -> Ccaller_DiagLv1/6(diagFaultCntThresh)
  diagPassCntThresh/1 -> Ccaller_DiagLv1/7(diagPassCntThresh)
  diagDbncEnab/1 -> Ccaller_DiagLv1/5(diagDbncEnable)
  diagReset/1 -> Ccaller_DiagLv1/3(diagReset)
  diagEnable/1 -> Ccaller_DiagLv1/4(diagEnable)
  diagHealEn/1 -> Ccaller_DiagLv1/10(diagHealEn)
  Ccaller_DiagLv1/1(diagFaultStatus) -> diagFaultStatus/1
  Ccaller_DiagLv1/2(diagFaultCnt) -> diagFaultCnt/1

== system common_lib/Diagnostics/DTNA_Diag/S_Diag ==
  diagInput : Inport
  diagStartUpComp : Inport  Port=2
  diagUpCnt : Inport  Port=3
  diagDnCnt : Inport  Port=4
  diagFaultCntThresh : Inport  Port=5
  diagPassCntThresh : Inport  Port=6
  diagDbncEnab : Inport  Port=7
  diagReset : Inport  Port=8
  diagEnable : Inport  Port=9
  diagHealEn : Inport  Port=10
  DiagFaultCounter : Subsystem
  diagFaultStatus : Outport  OutputWhenDisabled=reset  InitialOutput=Dem_EventStatusType.DEM_EVENT_STATUS_INIT  VectorParamsAs1DForOutWhenUnconnected=off
  diagFaultCnt : Outport  Port=2  OutputWhenDisabled=reset  InitialOutput=Dem_EventStatusType.DEM_EVENT_STATUS_INIT  VectorParamsAs1DForOutWhenUnconnected=off
  wires:
  diagHealEn/1 -> DiagFaultCounter/10(diagHealEn)
  diagPassCntThresh/1 -> DiagFaultCounter/7(diagPassCntThresh)
  diagInput/1 -> DiagFaultCounter/1(diagFaultActive)
  diagStartUpComp/1 -> DiagFaultCounter/2(diagStartUpComp)
  diagReset/1 -> DiagFaultCounter/3(diagReset)
  diagEnable/1 -> DiagFaultCounter/4(diagEnable)
  diagDbncEnab/1 -> DiagFaultCounter/5(diagDbncEnab)
  diagFaultCntThresh/1 -> DiagFaultCounter/6(diagFaultCntThresh)
  diagUpCnt/1 -> DiagFaultCounter/8(diagUpCnt)
  diagDnCnt/1 -> DiagFaultCounter/9(diagDnCnt)
  DiagFaultCounter/1(diagFaultStatus) -> diagFaultStatus/1
  DiagFaultCounter/2(diagFaultCnt) -> diagFaultCnt/1

== system common_lib/Diagnostics/SetFMI/IF_ELSE_LADDER ==
  FMI_in : Inport  OutDataTypeStr=uint8  PortDimensions=1
  Active1 : Inport  Port=2  OutDataTypeStr=boolean  PortDimensions=1
  Active2 : Inport  Port=3  OutDataTypeStr=boolean  PortDimensions=1
  Active3 : Inport  Port=4  OutDataTypeStr=boolean  PortDimensions=1
  Active4 : Inport  Port=5  OutDataTypeStr=boolean  PortDimensions=1
  Active5 : Inport  Port=6  OutDataTypeStr=boolean  PortDimensions=1
  Active6 : Inport  Port=7  OutDataTypeStr=boolean  PortDimensions=1
  Active7 : Inport  Port=8  OutDataTypeStr=boolean  PortDimensions=1
  FMI_1 : Inport  Port=9  OutDataTypeStr=uint8  PortDimensions=1
  FMI_2 : Inport  Port=10  OutDataTypeStr=uint8  PortDimensions=1
  FMI_3 : Inport  Port=11  OutDataTypeStr=uint8  PortDimensions=1
  FMI_4 : Inport  Port=12  OutDataTypeStr=uint8  PortDimensions=1
  FMI_5 : Inport  Port=13  OutDataTypeStr=uint8  PortDimensions=1
  FMI_6 : Inport  Port=14  OutDataTypeStr=uint8  PortDimensions=1
  FMI_7 : Inport  Port=15  OutDataTypeStr=uint8  PortDimensions=1
  Constant1 : Constant  Value=FMI32_NO_FAULT
  Constant7 : Constant  Value=FMI32_NO_FAULT
  Relational Operator : RelationalOperator  Operator=~=  OutDataTypeStr=boolean  RndMeth=Nearest
  Switch{,1..7} (8 alike) : Switch  Threshold=0.5
  FMI_out : Outport  OutDataTypeStr=uint8  PortDimensions=1  VectorParamsAs1DForOutWhenUnconnected=off
  wires:
  Constant1/1 -> Switch7/3
  FMI_in/1 -> Relational Operator/1, Switch/1
  Active6/1 -> Switch6/2
  Switch1/1 -> Switch/3
  FMI_2/1 -> Switch2/1
  Switch4/1 -> Switch3/3
  FMI_5/1 -> Switch5/1
  Switch3/1 -> Switch2/3
  Switch6/1 -> Switch5/3
  Switch/1 -> FMI_out/1
  FMI_4/1 -> Switch4/1
  FMI_7/1 -> Switch7/1
  FMI_3/1 -> Switch3/1
  Switch7/1 -> Switch6/3
  Active4/1 -> Switch4/2
  Switch5/1 -> Switch4/3
  Constant7/1 -> Relational Operator/2
  Switch2/1 -> Switch1/3
  Active2/1 -> Switch2/2
  Active7/1 -> Switch7/2
  Active1/1 -> Switch1/2
  Active3/1 -> Switch3/2
  Active5/1 -> Switch5/2
  FMI_6/1 -> Switch6/1
  FMI_1/1 -> Switch1/1
  Relational Operator/1 -> Switch/2

== system common_lib/Diagnostics/SignalSubstitution/If Action Subsystem ==
  NoSubstitute : Inport
  Action Port : ActionPort
  Constant4 : Constant  Value=QLTY_SIGNAL_FULLY_FUNCTION  SampleTime=-1
  Signal Conversion : SignalConversion  OverrideOpt=off
  Signal : Outport  VectorParamsAs1DForOutWhenUnconnected=off
  Qlty : Outport  Port=2  VectorParamsAs1DForOutWhenUnconnected=off
  wires:
  NoSubstitute/1 -> Signal Conversion/1
  Constant4/1 -> Qlty/1
  Signal Conversion/1 -> Signal/1

== system common_lib/Diagnostics/SignalSubstitution/If Action Subsystem1 ==
  FirstChoice : Inport
  Action Port : ActionPort
  Constant4 : Constant  Value=QLTY_SIGNAL_SUBSTITUTED_BY_1ST_CHOICE  SampleTime=-1
  Signal Conversion : SignalConversion  OverrideOpt=off
  Signal : Outport  VectorParamsAs1DForOutWhenUnconnected=off
  Qlty : Outport  Port=2  VectorParamsAs1DForOutWhenUnconnected=off
  wires:
  Constant4/1 -> Qlty/1
  FirstChoice/1 -> Signal Conversion/1
  Signal Conversion/1 -> Signal/1

== system common_lib/Diagnostics/SignalSubstitution/If Action Subsystem2 ==
  SecondChoice : Inport
  Action Port : ActionPort
  Constant4 : Constant  Value=QLTY_SIGNAL_SUBSTITUTED_BY_2ND_CHOICE  SampleTime=-1
  Signal Conversion : SignalConversion  OverrideOpt=off
  Signal : Outport  VectorParamsAs1DForOutWhenUnconnected=off
  Qlty : Outport  Port=2  VectorParamsAs1DForOutWhenUnconnected=off
  wires:
  Signal Conversion/1 -> Signal/1
  SecondChoice/1 -> Signal Conversion/1
  Constant4/1 -> Qlty/1

== system common_lib/Diagnostics/SignalSubstitution/If Action Subsystem3 ==
  ThirdChoice : Inport
  Action Port : ActionPort
  Constant4 : Constant  Value=QLTY_SIGNAL_SUBSTITUTED_BY_3RD_CHOICE  SampleTime=-1
  Signal Conversion : SignalConversion  OverrideOpt=off
  Signal : Outport  VectorParamsAs1DForOutWhenUnconnected=off
  Qlty : Outport  Port=2  VectorParamsAs1DForOutWhenUnconnected=off
  wires:
  Constant4/1 -> Qlty/1
  ThirdChoice/1 -> Signal Conversion/1
  Signal Conversion/1 -> Signal/1

== system common_lib/Diagnostics/SignalSubstitution/If Action Subsystem4 ==
  FourthChoice : Inport
  Action Port : ActionPort
  Constant4 : Constant  Value=QLTY_SIGNAL_SUBSTITUTED_BY_4TH_CHOICE  SampleTime=-1
  Signal Conversion : SignalConversion  OverrideOpt=off
  Signal : Outport  VectorParamsAs1DForOutWhenUnconnected=off
  Qlty : Outport  Port=2  VectorParamsAs1DForOutWhenUnconnected=off
  wires:
  Signal Conversion/1 -> Signal/1
  FourthChoice/1 -> Signal Conversion/1
  Constant4/1 -> Qlty/1

== system common_lib/Diagnostics/SignalSubstitution/If Action Subsystem5 ==
  FailedValue : Inport
  Action Port : ActionPort
  Constant4 : Constant  Value=QLTY_SIGNAL_FAILED  SampleTime=-1
  Signal Conversion : SignalConversion  OverrideOpt=off
  Signal : Outport  VectorParamsAs1DForOutWhenUnconnected=off
  Qlty : Outport  Port=2  VectorParamsAs1DForOutWhenUnconnected=off
  wires:
  Constant4/1 -> Qlty/1
  FailedValue/1 -> Signal Conversion/1
  Signal Conversion/1 -> Signal/1

== system common_lib/Fltrs/Fltr_wRO/FilterCoreLogic ==
  note: This is a simple 1st order filter block
  input : Inport  OutDataTypeStr=single
  tau : Inport  Port=2  OutDataTypeStr=single
  override_value : Inport  Port=3
  override? : Inport  Port=4  OutDataTypeStr=boolean
  reset? : Inport  Port=5  OutDataTypeStr=boolean
  Constant1 : Constant  Value=Ts
  MinMax : MinMax  Function=max  Inputs=2  InputSameDT=on  SaturateOnIntegerOverflow=on  ZeroCross=off
  Product : Product  Inputs=**/  InputSameDT=on  OutDataTypeStr=Inherit: Same as first input
  Sum : Sum  Inputs=|+-  InputSameDT=on  OutDataTypeStr=Inherit: Same as first input
  Sum1 : Sum  Inputs=|++  InputSameDT=on  OutDataTypeStr=Inherit: Same as first input
  Switch : Switch  Threshold=0.5  ZeroCross=off  InputSameDT=on
  Switch2 : Switch  Threshold=0.5  ZeroCross=off  InputSameDT=on
  Unit Delay : UnitDelay  InitialCondition=IC  SampleTime=-1  HasFrameUpgradeWarning=on
  output : Outport  OutDataTypeStr=single  VectorParamsAs1DForOutWhenUnconnected=off
  wires:
  Sum1/1 -> Switch2/3
  Product/1 -> Sum1/1
  tau/1 -> MinMax/2
  input/1 -> Sum/1, Switch2/1
  MinMax/1 -> Product/3
  Sum/1 -> Product/1
  Constant1/1 -> MinMax/1, Product/2
  override_value/1 -> Switch/1
  override?/1 -> Switch/2
  Switch/1 -> output/1, Unit Delay/1
  reset?/1 -> Switch2/2
  Switch2/1 -> Switch/3
  Unit Delay/1 -> Sum1/2, Sum/2

== system common_lib/Fltrs/Fltr_wROExtInitCond/FilterCoreLogic ==
  note: This is a simple 1st order filter block
  input : Inport  OutDataTypeStr=single
  tau : Inport  Port=2  OutDataTypeStr=single
  init_cond : Inport  Port=3  OutDataTypeStr=single
  task_rate : Inport  Port=4  OutDataTypeStr=single
  reset : Inport  Port=5  OutDataTypeStr=boolean
  override : Inport  Port=6  OutDataTypeStr=boolean
  override_value : Inport  Port=7
  ClampAboveZero : $bdroot/Misc/ClampAboveZero  Tol=single(1e-9)
      settings: AttributesFormatString=tol=%<Tol>
  Constant : Constant  Value=FALSE  SampleTime=-1
  MinMax : MinMax  Function=max  Inputs=2  InputSameDT=on  SaturateOnIntegerOverflow=on  ZeroCross=off
  Product : Product  Inputs=**/  InputSameDT=on  OutDataTypeStr=Inherit: Same as first input
  Sum : Sum  Inputs=|+-  InputSameDT=on  OutDataTypeStr=Inherit: Same as first input
  Sum1 : Sum  Inputs=|++  InputSameDT=on  OutDataTypeStr=Inherit: Same as first input
  Switch : Switch  Threshold=0.5  ZeroCross=off  InputSameDT=on
  Switch1 : Switch  Criteria=u2 ~= 0  Threshold=0.5  ZeroCross=off  InputSameDT=on
  Switch2 : Switch  Threshold=0.5  ZeroCross=off  InputSameDT=on
  Unit Delay : UnitDelay  InitialCondition=TRUE  SampleTime=-1  HasFrameUpgradeWarning=on
      settings: AttributesFormatString=ic=%<X0>
  Unit Delay1 : UnitDelay  InitialCondition=single(0)  SampleTime=-1  HasFrameUpgradeWarning=on
      settings: AttributesFormatString=ic=%<X0>
  output : Outport  OutDataTypeStr=single  VectorParamsAs1DForOutWhenUnconnected=off
  wires:
  Switch1/1 -> Sum1/2, Sum/2
  Sum1/1 -> Switch2/3
  Product/1 -> Sum1/1
  tau/1 -> MinMax/2
  input/1 -> Switch2/1, Sum/1
  MinMax/1 -> ClampAboveZero/1
  Sum/1 -> Product/1
  task_rate/1 -> Product/2, MinMax/1
  override_value/1 -> Switch/1
  override/1 -> Switch/2
  Switch/1 -> output/1
  reset/1 -> Switch2/2
  Switch2/1 -> Unit Delay1/1, Switch/3
  Constant/1 -> Unit Delay/1
  Unit Delay/1 -> Switch1/2
  init_cond/1 -> Switch1/1
  Unit Delay1/1 -> Switch1/3
  ClampAboveZero/1 -> Product/3

== system common_lib/Fltrs/Int16FIR/Accum ==
  Buf : Inport
  Constant : Constant  Value=int16(2*N-2)
  Constant1 : Constant  Value=int16(N-1)
  Data Type Conversion : DataTypeConversion  OutDataTypeStr=int32
  Data Type Conversion1 : DataTypeConversion  OutDataTypeStr=int32
  Demux : Demux  Outputs=2
  For Iterator : ForIterator  ResetStates=reset  IterationLimit=N-1  IndexMode=Zero-based  IterationVariableDataType=int16
  Mux : Mux  Inputs=2
  Product : Product  OutDataTypeStr=int32
  Selector : Selector  IndexMode=Zero-based  InputPortWidth=2*N  IndexOptions=Index vector (port)  Indices=[1 3]  OutputSizes=1
  Sum : Sum  Inputs=++|  AccumDataTypeStr=int32  OutDataTypeStr=int32
  Sum1 : Sum  Inputs=|+-
  Sum2 : Sum  Inputs=|+-
  Sum3 : Sum  Inputs=|+-
  Sum4 : Sum  Inputs=+++  AccumDataTypeStr=int32  OutDataTypeStr=int32
  Unit Delay : UnitDelay  SampleTime=-1  HasFrameUpgradeWarning=on
  Unit Delay1 : UnitDelay  SampleTime=-1  HasFrameUpgradeWarning=on
  Accel_Accum : Outport  VectorParamsAs1DForOutWhenUnconnected=off
  Mean_Accum : Outport  Port=2  VectorParamsAs1DForOutWhenUnconnected=off
  wires:
  Unit Delay1/1 -> Sum4/1
  Demux/1 -> Sum1/1, Sum4/2
  Sum4/1 -> Unit Delay1/1, Mean_Accum/1
  Data Type Conversion1/1 -> Product/1
  Data Type Conversion/1 -> Demux/1
  Sum3/1 -> Mux/2
  Product/1 -> Sum/2
  Sum2/1 -> Data Type Conversion1/1
  Constant1/1 -> Sum2/1
  Sum1/1 -> Product/2
  Demux/2 -> Sum4/3, Sum1/2
  Unit Delay/1 -> Sum/1
  Selector/1 -> Data Type Conversion/1
  Buf/1 -> Selector/1
  Mux/1 -> Selector/2
  Constant/1 -> Sum3/1
  For Iterator/1 -> Sum3/2, Mux/1, Sum2/2
  Sum/1 -> Unit Delay/1, Accel_Accum/1

== system common_lib/Gear Ratios/FindGearNumberByRatio/Timer1 ==
  In : Inport
  TriggerTime : Inport  Port=2
  Data Type Conversion : DataTypeConversion  OutDataTypeStr=single
  Discrete-Time Integrator : DiscreteIntegrator  gainval=single(1.0)  ExternalReset=falling  InitialCondition=single(0)  SampleTime=TimeStep  LimitOutput=on  ICPrevOutput=DiscIntNeverNeededParam  ICPrevScaledInput=DiscIntNeverNeededParam
  Relational Operator : RelationalOperator  Operator=>  OutDataTypeStr=boolean  RndMeth=Nearest
  Signal Specification : SignalSpecification  OutDataTypeStr=boolean
  Out : Outport  VectorParamsAs1DForOutWhenUnconnected=off
  wires:
  Relational Operator/1 -> Out/1
  TriggerTime/1 -> Relational Operator/2
  Discrete-Time Integrator/1 -> Relational Operator/1
  Data Type Conversion/1 -> Discrete-Time Integrator/1
  In/1 -> Signal Specification/1
  Signal Specification/1 -> Data Type Conversion/1, Discrete-Time Integrator/2

== system common_lib/Misc/EdgeTriggered Pulse w time/EdgeTriggeredPulseCoreLogic ==
  note: Initial Condition
  note: Common Library::Miscellaneous::Edge Triggered Pulse with Time
  input : Inport  OutDataTypeStr=boolean
  width : Inport  Port=2  OutDataTypeStr=single
  And : Logic
  Constant2 : Constant  Value=true
  Constant3 : Constant  Value=false
  Logical Operator1 : Logic  Operator=OR
  Not : Logic  Operator=NOT
  Relational Operator1 : RelationalOperator  Operator=>  ZeroCross=off  RndMeth=Nearest  InputSameDT=on
  Sample Rate : Constant  Value=Ts
  Sample Rate Half : Constant  Value=Ts_half
  Sum : Sum  Inputs=|++  InputSameDT=on  OutDataTypeStr=Inherit: Same as first input
  Sum1 : Sum  Inputs=-+|  InputSameDT=on  OutDataTypeStr=Inherit: Same as first input
  Switch : Switch  Threshold=0.5  ZeroCross=off  InputSameDT=on
  Switch1 : Switch  Threshold=0.5  ZeroCross=off  InputSameDT=on
  Switch2 : Switch  Threshold=0.5  ZeroCross=off  InputSameDT=on
  Unit Delay1 : UnitDelay  InitialCondition=true  SampleTime=-1  HasFrameUpgradeWarning=on
      settings: AttributesFormatString=ic=%<X0>
  Unit Delay2 : UnitDelay  InitialCondition=single(0)  SampleTime=-1  HasFrameUpgradeWarning=on
      settings: AttributesFormatString=ic=%<X0>
  Unit Delay4 : UnitDelay  InitialCondition=true  SampleTime=-1  HasFrameUpgradeWarning=on
      settings: AttributesFormatString=ic=%<X0>
  pulse : Outport  OutDataTypeStr=boolean  VectorParamsAs1DForOutWhenUnconnected=off
  wires:
  input/1 -> And/1, Unit Delay1/1
  Sample Rate/1 -> Switch/1, Sum/1
  Constant3/1 -> Switch2/1
  Unit Delay4/1 -> Logical Operator1/2, Switch2/3
  Switch2/1 -> Switch1/3
  Constant2/1 -> Switch1/1
  Switch1/1 -> Unit Delay4/1, pulse/1
  Relational Operator1/1 -> Switch1/2
  And/1 -> Switch2/2, Logical Operator1/1
  Logical Operator1/1 -> Switch/2
  Unit Delay2/1 -> Sum/2
  Sum/1 -> Switch/3
  Sum1/1 -> Relational Operator1/1
  Not/1 -> And/2
  Unit Delay1/1 -> Not/1
  Switch/1 -> Unit Delay2/1, Sum1/2
  width/1 -> Relational Operator1/2
  Sample Rate Half/1 -> Sum1/1

== system common_lib/Misc/Timeout Detection/TimeoutLogic ==
  Change : Inport
  Timeout : Inport  Port=2
  MinMax : MinMax  Inputs=2  InputSameDT=on  SaturateOnIntegerOverflow=on  ZeroCross=off
  Sample Rate : Constant  Value=Ts
  Sample Rate Tolerance : Constant  Value=Tol
  Sum : Sum  Inputs=++|  InputSameDT=on  OutDataTypeStr=Inherit: Same as first input
  Sum1 : Sum  Inputs=-+|  InputSameDT=on  OutDataTypeStr=Inherit: Same as first input
  Switch : Switch  Threshold=0.5  ZeroCross=off  InputSameDT=on
  Unit Delay : UnitDelay  InitialCondition=Zero  SampleTime=-1  HasFrameUpgradeWarning=on
  zero : Constant  Value=Zero
  time : Outport  VectorParamsAs1DForOutWhenUnconnected=off
  wires:
  Unit Delay/1 -> Sum/1
  MinMax/1 -> Unit Delay/1
  zero/1 -> Switch/3
  Switch/1 -> Sum1/2, MinMax/2
  Sum/1 -> Switch/1
  Timeout/1 -> MinMax/1
  Sample Rate/1 -> Sum/2
  Sample Rate Tolerance/1 -> Sum1/1
  Sum1/1 -> time/1
  Change/1 -> Switch/2

== system common_lib/Misc/Timeout with time/TimeoutLogic ==
  Change : Inport
  Timeout : Inport  Port=2
  MinMax : MinMax  Inputs=2  InputSameDT=on  SaturateOnIntegerOverflow=on  ZeroCross=off
  Sample Rate : Constant  Value=Ts
  Sample Rate Tolerance : Constant  Value=Tol
  Sum : Sum  Inputs=++|  InputSameDT=on  OutDataTypeStr=Inherit: Same as first input
  Sum1 : Sum  Inputs=-+|  InputSameDT=on  OutDataTypeStr=Inherit: Same as first input
  Switch : Switch  Threshold=0.5  ZeroCross=off  InputSameDT=on
  Unit Delay : UnitDelay  InitialCondition=Zero  SampleTime=-1  HasFrameUpgradeWarning=on
  zero : Constant  Value=Zero
  time : Outport  VectorParamsAs1DForOutWhenUnconnected=off
  wires:
  Change/1 -> Switch/2
  Sum1/1 -> time/1
  Sample Rate Tolerance/1 -> Sum1/1
  Sample Rate/1 -> Sum/2
  Timeout/1 -> MinMax/1
  Sum/1 -> Switch/1
  Switch/1 -> MinMax/2, Sum1/2
  zero/1 -> Switch/3
  MinMax/1 -> Unit Delay/1
  Unit Delay/1 -> Sum/1

== system common_lib/OS/Scheduler with Init/Init Relay ==
  Task 1 : TriggerPort  TriggerType=function-call  VariantControl=(inherit)  StatesWhenEnabling=reset  ZeroCross=off
  Constant2 : Constant  Value=FALSE
  Function Call : Subsystem  TreatAsAtomicUnit=on
  Unit Delay2 : UnitDelay  InitialCondition=TRUE  SampleTime=-1  HasFrameUpgradeWarning=on
      settings: AttributesFormatString=ic=%<X0>
  Init : Outport  VectorParamsAs1DForOutWhenUnconnected=off
  wires:
  Function Call/1(Init) -> Init/1
  Constant2/1 -> Unit Delay2/1
  Unit Delay2/1 -> Function Call/Enable
